simulink model "LQR_test"  (R2023a)
settings: Solver=FixedStepDiscrete  StartTime=0.0  StopTime=input_settings.flight_time  FixedStep=input_settings.dt  RelTol=1e-3
undefined symbols (not defined in the file): DiscIntNeverNeededParam, input_settings, linear_sys, LQR_gain, saturation_deflection_rate
settings Model: Creator=sjd320  LastModifiedBy=sduess
settings DebuggingCC: UnconnectedInputMsg=warning  UnconnectedOutputMsg=warning  UnconnectedLineMsg=warning
settings ModelReferenceCC: EnableRefExpFcnMdlSchedulingChecks=on
settings RTWCC: DLArmComputeVersion=19.05

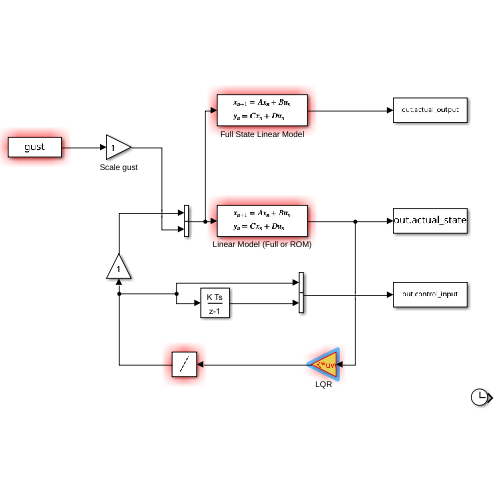
[thumbnail: Simulink's stored preview of the top-level diagram]
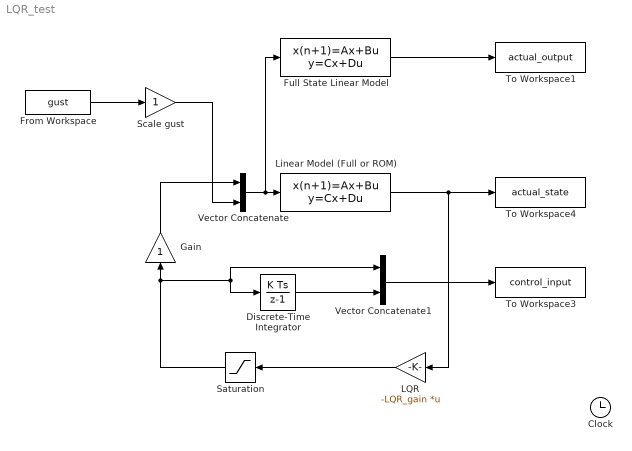
== system LQR_test ==
  Clock : Clock
  Discrete-Time Integrator : DiscreteIntegrator  SampleTime=-1  ICPrevOutput=DiscIntNeverNeededParam  ICPrevScaledInput=DiscIntNeverNeededParam
  From Workspace : FromWorkspace  VariableName=gust  SampleTime=-1
  Full State Linear Model : DiscreteStateSpace  A=linear_sys.A  B=linear_sys.B  C=linear_sys.C  D=linear_sys.D  SampleTime=input_settings.dt
  Gain : Gain
  LQR : Gain  Gain=-LQR_gain  Multiplication=Matrix(K*u) (u vector)
  Linear Model (Full or ROM) : DiscreteStateSpace  A=linear_sys.A  B=linear_sys.B  C=eye(size(linear_sys.A,1))  D=linear_sys.B .* 0.  SampleTime=input_settings.dt
  Saturation : Saturate  UpperLimit=saturation_deflection_rate  LowerLimit=-saturation_deflection_rate
  Scale gust : Gain
  To Workspace1 : ToWorkspace  VariableName=actual_output  SaveFormat=Timeseries  SampleTime=-1
  To Workspace3 : ToWorkspace  VariableName=control_input  SaveFormat=Timeseries  SampleTime=-1
  To Workspace4 : ToWorkspace  VariableName=actual_state  SaveFormat=Timeseries  SampleTime=-1
  Vector Concatenate : Concatenate
  Vector Concatenate1 : Concatenate
  wires:
  Vector Concatenate/1 -> Full State Linear Model/1, Linear Model (Full or ROM)/1
  From Workspace/1 -> Scale gust/1
  Scale gust/1 -> Vector Concatenate/2
  Full State Linear Model/1 -> To Workspace1/1
  Linear Model (Full or ROM)/1 -> LQR/1, To Workspace4/1
  LQR/1 -> Saturation/1
  Saturation/1 -> Vector Concatenate1/1, Discrete-Time Integrator/1, Gain/1
  Gain/1 -> Vector Concatenate/1
  Vector Concatenate1/1 -> To Workspace3/1
  Discrete-Time Integrator/1 -> Vector Concatenate1/2
